simulink model "week3_2"  (R2020b)
settings: Solver=VariableStepAuto  StartTime=0.0  StopTime=10.0  RelTol=1e-3
settings Model: Creator=lalit  LastModifiedBy=lalit

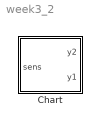
== system week3_2 ==
  Chart : Stateflow chart  TreatAsAtomicUnit=on

== stateflow chart week3_2/Chart ==
  state prep_to_stop
    y1 = R;
    y2 = G ;
  state StopToGo
    y1 = R;
    y2 = Y;
  state Redlight
    y1=R;
    y2=G;
  state Go
    y1 = G;
    y2 = R;
  state GoToStop
    y1 = Y;
    y2 = R;
  (default) -> Redlight
  Redlight -> prep_to_stop : after(20,tick)
  prep_to_stop -> StopToGo : [sens]
  StopToGo -> Go : after(3,tick)
  GoToStop -> Redlight : after(3,tick)
  Go -> GoToStop : after(10,tick)
  data: sens input; y2 output; y1 output; R constant double size=1; G constant double size=3; Y constant double size=2
